simulink model "Computer"  (R2023a)
settings: Solver=VariableStepDiscrete  StartTime=0.0  StopTime=inf  RelTol=1e-3  EnableMultiTasking=on
values from neighbouring files (symbols this model uses):
  RomCode = Preprocessor(RomCode, c)    [ROM.m]
undefined symbols (not defined in the file or in its folder): c, in, RomCodeBreakpoints, RomData, RomDataBreakpoints, UartDataRx, UartDataRx_Active
libraries: Miscellaneous x281, simulink_extras x66, Memory_Blocks_Lib x46, simulink x42, Word_Multiplexers_Lib x31, Decoders_Lib x30, Encoders_Lib x10, Counters_Lib x9, Bit_Multiplexers_Lib x8, Arithmetic_Operations_Lib x5, Bit_Demultiplexers_Lib x4, Garbage x1
(part 5 of 6)

== system Computer/Register Debug ==
  In8 : Inport
  In7 : Inport  Port=2
  In6 : Inport  Port=3
  In5 : Inport  Port=4
  In4 : Inport  Port=5
  In3 : Inport  Port=6
  In2 : Inport  Port=7
  In1 : Inport  Port=8
  Bit to Integer Converter{1..8} (8 alike) : simulink/Logic and Bit Operations/Bit to Integer Converter  nbits=16  bitOrder=MSB first  signedOutputValues=Unsigned  outDtype=uint16  outDtypeSigned=Inherit via internal rule
      settings: LibrarySourceBlock=|
      | commutil2/Bit to Integer
      | Converter
  To Workspace : ToWorkspace  VariableName=gp_reg_00  SampleTime=-1
      settings: MaxDataPoints=1  Save2DSignal=2-D array (concatenate along first dimension)
  To Workspace1 : ToWorkspace  VariableName=gp_reg_01  SampleTime=-1
      settings: MaxDataPoints=1  Save2DSignal=2-D array (concatenate along first dimension)
  To Workspace2 : ToWorkspace  VariableName=gp_reg_02  SampleTime=-1
      settings: MaxDataPoints=1  Save2DSignal=2-D array (concatenate along first dimension)
  To Workspace3 : ToWorkspace  VariableName=gp_reg_03  SampleTime=-1
      settings: MaxDataPoints=1  Save2DSignal=2-D array (concatenate along first dimension)
  To Workspace4 : ToWorkspace  VariableName=gp_reg_04  SampleTime=-1
      settings: MaxDataPoints=1  Save2DSignal=2-D array (concatenate along first dimension)
  To Workspace5 : ToWorkspace  VariableName=gp_reg_05  SampleTime=-1
      settings: MaxDataPoints=1  Save2DSignal=2-D array (concatenate along first dimension)
  To Workspace6 : ToWorkspace  VariableName=gp_reg_06  SampleTime=-1
      settings: MaxDataPoints=1  Save2DSignal=2-D array (concatenate along first dimension)
  To Workspace7 : ToWorkspace  VariableName=gp_reg_07  SampleTime=-1
      settings: MaxDataPoints=1  Save2DSignal=2-D array (concatenate along first dimension)
  wires:
  Bit to Integer Converter1/1 -> To Workspace1/1
  Bit to Integer Converter3/1 -> To Workspace3/1
  Bit to Integer Converter7/1 -> To Workspace7/1
  In8/1 -> Bit to Integer Converter8/1
  Bit to Integer Converter4/1 -> To Workspace4/1
  Bit to Integer Converter5/1 -> To Workspace5/1
  Bit to Integer Converter2/1 -> To Workspace2/1
  Bit to Integer Converter8/1 -> To Workspace/1
  Bit to Integer Converter6/1 -> To Workspace6/1
  In6/1 -> Bit to Integer Converter2/1
  In2/1 -> Bit to Integer Converter6/1
  In5/1 -> Bit to Integer Converter3/1
  In4/1 -> Bit to Integer Converter4/1
  In7/1 -> Bit to Integer Converter1/1
  In1/1 -> Bit to Integer Converter7/1
  In3/1 -> Bit to Integer Converter5/1

== system Computer/Screen_40x25 ==
  Data(1000B) : Inport
  Byte_2 : Constant  Value=c.char_7x7(:, :, 1:256)  OutDataTypeStr=uint8
  MATLAB Function : MATLAB Function  TreatAsAtomicUnit=on
  Matrix Viewer1 : dspobslib/Matrix Viewer  ImageParams=off  CMapStr=[0 0.3 0; 0 1 0]  AxisColorbar=on  AxisParams=off  AxisOrigin=Upper left corner  AxisTickMode=Auto  XTickRange=[0 1]  YTickRange=[0 1]  XLabel=X-axis  YLabel=Y-axis  ZLabel=Z-axis  FigPos=[1280 555 320*2 246*2]  AxisZoom=on
      settings: YMin=0  YMax=1
  wires:
  MATLAB Function/1(Framebuffer) -> Matrix Viewer1/1
  Data(1000B)/1 -> MATLAB Function/2(VideoMemory)
  Byte_2/1 -> MATLAB Function/1(CharTable)

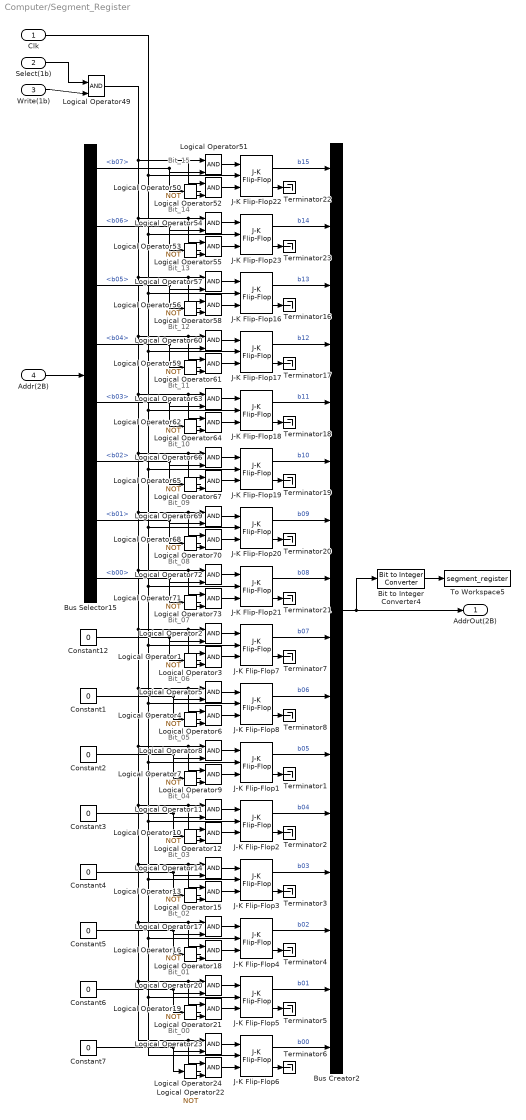
== system Computer/Segment_Register ==
  note: Bit_00
  note: Bit_01
  note: Bit_02
  note: Bit_03
  note: Bit_04
  note: Bit_05
  note: Bit_06
  note: Bit_07
  note: Bit_08
  note: Bit_09
  note: Bit_10
  note: Bit_11
  note: Bit_12
  note: Bit_13
  note: Bit_14
  note: Bit_15
  Clk : Inport  OutDataTypeStr=double
  Select(1b) : Inport  Port=2
  Write(1b) : Inport  Port=3
  Addr(2B) : Inport  Port=4
  Bit to Integer Converter4 : simulink/Logic and Bit Operations/Bit to Integer Converter  nbits=16  bitOrder=MSB first  signedOutputValues=Unsigned  outDtype=uint16  outDtypeSigned=Inherit via internal rule
      settings: LibrarySourceBlock=|
      | commutil2/Bit to Integer
      | Converter
  Bus Creator2 : BusCreator  Inputs=16
  Bus Selector15 : BusSelector  OutputSignals=b07,b06,b05,b04,b03,b02,b01,b00
  Constant{1..7,12} (8 alike) : Constant  Value=0  OutDataTypeStr=boolean
  J-K Flip-Flop{1..8,16..23} (16 alike) : simulink_extras/Flip Flops/J-K Flip-Flop  initial_condition=0
  Logical Operator{1,4,7,10,13,16,19,22,50,53,56,59,62,65,68,71} (16 alike) : Logic  Operator=NOT  IconShape=distinctive  AllPortsSameDT=off  OutDataTypeStr=boolean
  Logical Operator{2..3,5..6,8..9,11..12,14..15,17..18,20..21,23..24,49,51..52,54..55,57..58,60..61,63..64,66..67,69..70,72..73} (33 alike) : Logic  IconShape=distinctive  AllPortsSameDT=off  OutDataTypeStr=boolean
  Terminator{1..8,16..23} (16 alike) : Terminator
  To Workspace5 : ToWorkspace  VariableName=segment_register  SampleTime=-1
      settings: MaxDataPoints=1  Save2DSignal=2-D array (concatenate along first dimension)
  AddrOut(2B) : Outport
  wires:
  J-K Flip-Flop6/2 -> Terminator6/1
  J-K Flip-Flop6/1 -> Bus Creator2/16  "b00"
  Logical Operator22/1 -> Logical Operator24/2
  Logical Operator23/1 -> J-K Flip-Flop6/1
  Logical Operator24/1 -> J-K Flip-Flop6/3
  J-K Flip-Flop5/2 -> Terminator5/1
  J-K Flip-Flop5/1 -> Bus Creator2/15  "b01"
  Logical Operator49/1 -> Logical Operator52/1, Logical Operator51/1, Logical Operator72/1, Logical Operator73/1, Logical Operator20/1, Logical Operator21/1, Logical Operator23/1, Logical Operator24/1, Logical Operator17/1, Logical Operator18/1, Logical Operator14/1, Logical Operator15/1, Logical Operator11/1, Logical Operator12/1, Logical Operator8/1, Logical Operator9/1, Logical Operator5/1, Logical Operator6/1, Logical Operator3/1, Logical Operator2/1, Logical Operator69/1, Logical Operator70/1, Logical Operator66/1, Logical Operator67/1, Logical Operator63/1, Logical Operator64/1, Logical Operator60/1, Logical Operator61/1, Logical Operator57/1, Logical Operator58/1, Logical Operator54/1, Logical Operator55/1
  Logical Operator19/1 -> Logical Operator21/2
  Logical Operator20/1 -> J-K Flip-Flop5/1
  Logical Operator21/1 -> J-K Flip-Flop5/3
  J-K Flip-Flop4/2 -> Terminator4/1
  J-K Flip-Flop4/1 -> Bus Creator2/14  "b02"
  Logical Operator16/1 -> Logical Operator18/2
  Logical Operator17/1 -> J-K Flip-Flop4/1
  Logical Operator18/1 -> J-K Flip-Flop4/3
  J-K Flip-Flop3/2 -> Terminator3/1
  J-K Flip-Flop3/1 -> Bus Creator2/13  "b03"
  Logical Operator13/1 -> Logical Operator15/2
  Logical Operator14/1 -> J-K Flip-Flop3/1
  Logical Operator15/1 -> J-K Flip-Flop3/3
  J-K Flip-Flop2/2 -> Terminator2/1
  J-K Flip-Flop2/1 -> Bus Creator2/12  "b04"
  Logical Operator10/1 -> Logical Operator12/2
  Logical Operator11/1 -> J-K Flip-Flop2/1
  Logical Operator12/1 -> J-K Flip-Flop2/3
  J-K Flip-Flop1/2 -> Terminator1/1
  J-K Flip-Flop1/1 -> Bus Creator2/11  "b05"
  Clk/1 -> J-K Flip-Flop22/2, J-K Flip-Flop23/2, J-K Flip-Flop16/2, J-K Flip-Flop17/2, J-K Flip-Flop18/2, J-K Flip-Flop19/2, J-K Flip-Flop20/2, J-K Flip-Flop21/2, J-K Flip-Flop7/2, J-K Flip-Flop8/2, J-K Flip-Flop2/2, J-K Flip-Flop3/2, J-K Flip-Flop4/2, J-K Flip-Flop5/2, J-K Flip-Flop6/2, J-K Flip-Flop1/2
  Logical Operator7/1 -> Logical Operator9/2
  Logical Operator8/1 -> J-K Flip-Flop1/1
  Logical Operator9/1 -> J-K Flip-Flop1/3
  J-K Flip-Flop8/2 -> Terminator8/1
  J-K Flip-Flop8/1 -> Bus Creator2/10  "b06"
  Logical Operator4/1 -> Logical Operator6/2
  Logical Operator5/1 -> J-K Flip-Flop8/1
  Logical Operator6/1 -> J-K Flip-Flop8/3
  J-K Flip-Flop7/2 -> Terminator7/1
  J-K Flip-Flop7/1 -> Bus Creator2/9  "b07"
  Logical Operator1/1 -> Logical Operator3/2
  Logical Operator2/1 -> J-K Flip-Flop7/1
  Logical Operator3/1 -> J-K Flip-Flop7/3
  Bus Selector15/1 -> Logical Operator50/1, Logical Operator51/2  "<b07>"
  Bus Selector15/8 -> Logical Operator72/2, Logical Operator71/1  "<b00>"
  J-K Flip-Flop21/2 -> Terminator21/1
  J-K Flip-Flop21/1 -> Bus Creator2/8  "b08"
  Logical Operator71/1 -> Logical Operator73/2
  Logical Operator72/1 -> J-K Flip-Flop21/1
  Logical Operator73/1 -> J-K Flip-Flop21/3
  Bus Selector15/7 -> Logical Operator69/2, Logical Operator68/1  "<b01>"
  J-K Flip-Flop20/2 -> Terminator20/1
  J-K Flip-Flop20/1 -> Bus Creator2/7  "b09"
  Logical Operator68/1 -> Logical Operator70/2
  Logical Operator69/1 -> J-K Flip-Flop20/1
  Logical Operator70/1 -> J-K Flip-Flop20/3
  Bus Selector15/6 -> Logical Operator66/2, Logical Operator65/1  "<b02>"
  J-K Flip-Flop19/2 -> Terminator19/1
  J-K Flip-Flop19/1 -> Bus Creator2/6  "b10"
  Logical Operator65/1 -> Logical Operator67/2
  Logical Operator66/1 -> J-K Flip-Flop19/1
  Logical Operator67/1 -> J-K Flip-Flop19/3
  Bus Selector15/5 -> Logical Operator63/2, Logical Operator62/1  "<b03>"
  J-K Flip-Flop18/2 -> Terminator18/1
  J-K Flip-Flop18/1 -> Bus Creator2/5  "b11"
  Logical Operator62/1 -> Logical Operator64/2
  Logical Operator63/1 -> J-K Flip-Flop18/1
  Logical Operator64/1 -> J-K Flip-Flop18/3
  Bus Selector15/4 -> Logical Operator60/2, Logical Operator59/1  "<b04>"
  J-K Flip-Flop17/2 -> Terminator17/1
  J-K Flip-Flop17/1 -> Bus Creator2/4  "b12"
  Logical Operator59/1 -> Logical Operator61/2
  Logical Operator60/1 -> J-K Flip-Flop17/1
  Logical Operator61/1 -> J-K Flip-Flop17/3
  Bus Selector15/3 -> Logical Operator57/2, Logical Operator56/1  "<b05>"
  J-K Flip-Flop16/2 -> Terminator16/1
  J-K Flip-Flop16/1 -> Bus Creator2/3  "b13"
  Logical Operator56/1 -> Logical Operator58/2
  Logical Operator57/1 -> J-K Flip-Flop16/1
  Logical Operator58/1 -> J-K Flip-Flop16/3
  Bus Selector15/2 -> Logical Operator53/1, Logical Operator54/2  "<b06>"
  J-K Flip-Flop23/2 -> Terminator23/1
  J-K Flip-Flop23/1 -> Bus Creator2/2  "b14"
  Logical Operator53/1 -> Logical Operator55/2
  Logical Operator54/1 -> J-K Flip-Flop23/1
  Logical Operator55/1 -> J-K Flip-Flop23/3
  J-K Flip-Flop22/2 -> Terminator22/1
  J-K Flip-Flop22/1 -> Bus Creator2/1  "b15"
  Logical Operator50/1 -> Logical Operator52/2
  Logical Operator51/1 -> J-K Flip-Flop22/1
  Logical Operator52/1 -> J-K Flip-Flop22/3
  Addr(2B)/1 -> Bus Selector15/1
  Select(1b)/1 -> Logical Operator49/1
  Write(1b)/1 -> Logical Operator49/2
  Bus Creator2/1 -> Bit to Integer Converter4/1, AddrOut(2B)/1
  Bit to Integer Converter4/1 -> To Workspace5/1
  Constant12/1 -> Logical Operator1/1, Logical Operator2/2
  Constant1/1 -> Logical Operator4/1, Logical Operator5/2
  Constant2/1 -> Logical Operator8/2, Logical Operator7/1
  Constant3/1 -> Logical Operator10/1, Logical Operator11/2
  Constant4/1 -> Logical Operator13/1, Logical Operator14/2
  Constant5/1 -> Logical Operator17/2, Logical Operator16/1
  Constant6/1 -> Logical Operator20/2, Logical Operator19/1
  Constant7/1 -> Logical Operator22/1, Logical Operator23/2

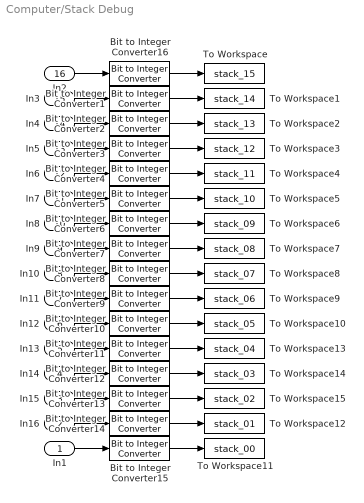
== system Computer/Stack Debug ==
  In1 : Inport
  In16 : Inport  Port=2
  In15 : Inport  Port=3
  In14 : Inport  Port=4
  In13 : Inport  Port=5
  In12 : Inport  Port=6
  In11 : Inport  Port=7
  In10 : Inport  Port=8
  In9 : Inport  Port=9
  In8 : Inport  Port=10
  In7 : Inport  Port=11
  In6 : Inport  Port=12
  In5 : Inport  Port=13
  In4 : Inport  Port=14
  In3 : Inport  Port=15
  In2 : Inport  Port=16
  Bit to Integer Converter{1..16} (16 alike) : simulink/Logic and Bit Operations/Bit to Integer Converter  nbits=16  bitOrder=MSB first  signedOutputValues=Unsigned  outDtype=uint16  outDtypeSigned=Inherit via internal rule
      settings: LibrarySourceBlock=|
      | commutil2/Bit to Integer
      | Converter
  To Workspace : ToWorkspace  VariableName=stack_15  SampleTime=-1
      settings: MaxDataPoints=1  Save2DSignal=2-D array (concatenate along first dimension)
  To Workspace1 : ToWorkspace  VariableName=stack_14  SampleTime=-1
      settings: MaxDataPoints=1  Save2DSignal=2-D array (concatenate along first dimension)
  To Workspace10 : ToWorkspace  VariableName=stack_05  SampleTime=-1
      settings: MaxDataPoints=1  Save2DSignal=2-D array (concatenate along first dimension)
  To Workspace11 : ToWorkspace  VariableName=stack_00  SampleTime=-1
      settings: MaxDataPoints=1  Save2DSignal=2-D array (concatenate along first dimension)
  To Workspace12 : ToWorkspace  VariableName=stack_01  SampleTime=-1
      settings: MaxDataPoints=1  Save2DSignal=2-D array (concatenate along first dimension)
  To Workspace13 : ToWorkspace  VariableName=stack_04  SampleTime=-1
      settings: MaxDataPoints=1  Save2DSignal=2-D array (concatenate along first dimension)
  To Workspace14 : ToWorkspace  VariableName=stack_03  SampleTime=-1
      settings: MaxDataPoints=1  Save2DSignal=2-D array (concatenate along first dimension)
  To Workspace15 : ToWorkspace  VariableName=stack_02  SampleTime=-1
      settings: MaxDataPoints=1  Save2DSignal=2-D array (concatenate along first dimension)
  To Workspace2 : ToWorkspace  VariableName=stack_13  SampleTime=-1
      settings: MaxDataPoints=1  Save2DSignal=2-D array (concatenate along first dimension)
  To Workspace3 : ToWorkspace  VariableName=stack_12  SampleTime=-1
      settings: MaxDataPoints=1  Save2DSignal=2-D array (concatenate along first dimension)
  To Workspace4 : ToWorkspace  VariableName=stack_11  SampleTime=-1
      settings: MaxDataPoints=1  Save2DSignal=2-D array (concatenate along first dimension)
  To Workspace5 : ToWorkspace  VariableName=stack_10  SampleTime=-1
      settings: MaxDataPoints=1  Save2DSignal=2-D array (concatenate along first dimension)
  To Workspace6 : ToWorkspace  VariableName=stack_09  SampleTime=-1
      settings: MaxDataPoints=1  Save2DSignal=2-D array (concatenate along first dimension)
  To Workspace7 : ToWorkspace  VariableName=stack_08  SampleTime=-1
      settings: MaxDataPoints=1  Save2DSignal=2-D array (concatenate along first dimension)
  To Workspace8 : ToWorkspace  VariableName=stack_07  SampleTime=-1
      settings: MaxDataPoints=1  Save2DSignal=2-D array (concatenate along first dimension)
  To Workspace9 : ToWorkspace  VariableName=stack_06  SampleTime=-1
      settings: MaxDataPoints=1  Save2DSignal=2-D array (concatenate along first dimension)
  wires:
  Bit to Integer Converter8/1 -> To Workspace8/1
  Bit to Integer Converter2/1 -> To Workspace2/1
  Bit to Integer Converter13/1 -> To Workspace15/1
  In5/1 -> Bit to Integer Converter3/1
  Bit to Integer Converter3/1 -> To Workspace3/1
  Bit to Integer Converter6/1 -> To Workspace6/1
  In3/1 -> Bit to Integer Converter1/1
  Bit to Integer Converter12/1 -> To Workspace14/1
  Bit to Integer Converter5/1 -> To Workspace5/1
  Bit to Integer Converter15/1 -> To Workspace11/1
  Bit to Integer Converter11/1 -> To Workspace13/1
  In16/1 -> Bit to Integer Converter14/1
  Bit to Integer Converter10/1 -> To Workspace10/1
  Bit to Integer Converter7/1 -> To Workspace7/1
  Bit to Integer Converter14/1 -> To Workspace12/1
  In10/1 -> Bit to Integer Converter8/1
  Bit to Integer Converter9/1 -> To Workspace9/1
  Bit to Integer Converter4/1 -> To Workspace4/1
  Bit to Integer Converter16/1 -> To Workspace/1
  Bit to Integer Converter1/1 -> To Workspace1/1
  In9/1 -> Bit to Integer Converter7/1
  In11/1 -> Bit to Integer Converter9/1
  In12/1 -> Bit to Integer Converter10/1
  In13/1 -> Bit to Integer Converter11/1
  In14/1 -> Bit to Integer Converter12/1
  In1/1 -> Bit to Integer Converter15/1
  In8/1 -> Bit to Integer Converter6/1
  In7/1 -> Bit to Integer Converter5/1
  In6/1 -> Bit to Integer Converter4/1
  In15/1 -> Bit to Integer Converter13/1
  In2/1 -> Bit to Integer Converter16/1
  In4/1 -> Bit to Integer Converter2/1

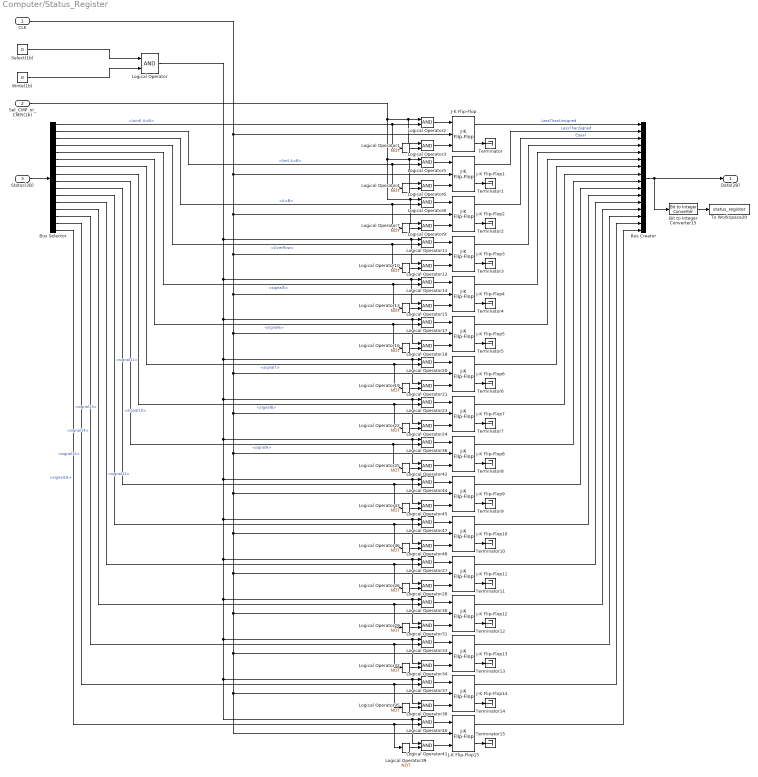
== system Computer/Status_Register ==
  CLK : Inport  OutDataTypeStr=double
  Sel_CMP_or_CMPI(1b) : Inport  Port=2
  Status(2B) : Inport  Port=3
  Bit to Integer Converter15 : simulink/Logic and Bit Operations/Bit to Integer Converter  nbits=16  bitOrder=MSB first  signedOutputValues=Unsigned  outDtype=uint16  outDtypeSigned=Inherit via internal rule
      settings: LibrarySourceBlock=|
      | commutil2/Bit to Integer
      | Converter
  Bus Creator : BusCreator  Inputs=16
  Bus Selector : BusSelector  OutputSignals=(uint) A<B,(int) A<B,A=B,Overflow,signal5,signal6,signal7,signal8,signal9,signal10,signal11,signal12,signal13,signal14,signal15,signal16
  J-K Flip-Flop{,1..15} (16 alike) : simulink_extras/Flip Flops/J-K Flip-Flop  initial_condition=0
  Logical Operator{,2..3,5..6,8..9,11..12,14..15,17..18,20..21,23..24,27..28,30..31,33..34,36..38,40..42,44..45,47..48} (33 alike) : Logic  IconShape=distinctive  AllPortsSameDT=off  OutDataTypeStr=boolean
  Logical Operator{1,4,7,10,13,16,19,22,25..26,29,32,35,39,43,46} (16 alike) : Logic  Operator=NOT  IconShape=distinctive  AllPortsSameDT=off  OutDataTypeStr=boolean
  Select(1b) : Constant  Value=0  OutDataTypeStr=boolean
  Terminator{,1..15} (16 alike) : Terminator
  To Workspace20 : ToWorkspace  VariableName=status_register  SampleTime=-1
      settings: MaxDataPoints=1  Save2DSignal=2-D array (concatenate along first dimension)
  Write(1b) : Constant  Value=0  OutDataTypeStr=boolean
  Data(2B) : Outport
  wires:
  Logical Operator41/1 -> J-K Flip-Flop15/3
  Logical Operator40/1 -> J-K Flip-Flop15/1
  Logical Operator39/1 -> Logical Operator41/2
  Logical Operator/1 -> Logical Operator11/1, Logical Operator12/1, Logical Operator14/1, Logical Operator15/1, Logical Operator18/1, Logical Operator17/1, Logical Operator20/1, Logical Operator21/1, Logical Operator23/1, Logical Operator24/1, Logical Operator36/1, Logical Operator42/1, Logical Operator44/1, Logical Operator45/1, Logical Operator47/1, Logical Operator48/1, Logical Operator27/1, Logical Operator28/1, Logical Operator30/1, Logical Operator31/1, Logical Operator34/1, Logical Operator33/1, Logical Operator37/1, Logical Operator38/1, Logical Operator40/1, Logical Operator41/1
  CLK/1 -> J-K Flip-Flop/2, J-K Flip-Flop1/2, J-K Flip-Flop2/2, J-K Flip-Flop3/2, J-K Flip-Flop4/2, J-K Flip-Flop5/2, J-K Flip-Flop7/2, J-K Flip-Flop8/2, J-K Flip-Flop9/2, J-K Flip-Flop10/2, J-K Flip-Flop11/2, J-K Flip-Flop12/2, J-K Flip-Flop13/2, J-K Flip-Flop15/2, J-K Flip-Flop14/2, J-K Flip-Flop6/2
  J-K Flip-Flop15/2 -> Terminator15/1
  Bus Selector/16 -> Logical Operator40/2, Logical Operator39/1  "<signal16>"
  Logical Operator38/1 -> J-K Flip-Flop14/3
  Logical Operator37/1 -> J-K Flip-Flop14/1
  Logical Operator35/1 -> Logical Operator38/2
  J-K Flip-Flop14/2 -> Terminator14/1
  Bus Selector/15 -> Logical Operator37/2, Logical Operator35/1  "<signal15>"
  Logical Operator34/1 -> J-K Flip-Flop13/3
  Logical Operator33/1 -> J-K Flip-Flop13/1
  Logical Operator32/1 -> Logical Operator34/2
  J-K Flip-Flop13/2 -> Terminator13/1
  Bus Selector/14 -> Logical Operator32/1, Logical Operator33/2  "<signal14>"
  Logical Operator31/1 -> J-K Flip-Flop12/3
  Logical Operator30/1 -> J-K Flip-Flop12/1
  Logical Operator29/1 -> Logical Operator31/2
  J-K Flip-Flop12/2 -> Terminator12/1
  Bus Selector/13 -> Logical Operator30/2, Logical Operator29/1  "<signal13>"
  Logical Operator28/1 -> J-K Flip-Flop11/3
  Logical Operator27/1 -> J-K Flip-Flop11/1
  Logical Operator26/1 -> Logical Operator28/2
  J-K Flip-Flop11/2 -> Terminator11/1
  Bus Selector/12 -> Logical Operator26/1, Logical Operator27/2  "<signal12>"
  Logical Operator48/1 -> J-K Flip-Flop10/3
  Logical Operator47/1 -> J-K Flip-Flop10/1
  Logical Operator46/1 -> Logical Operator48/2
  J-K Flip-Flop10/2 -> Terminator10/1
  Bus Selector/11 -> Logical Operator47/2, Logical Operator46/1  "<signal11>"
  Logical Operator45/1 -> J-K Flip-Flop9/3
  Logical Operator44/1 -> J-K Flip-Flop9/1
  Logical Operator43/1 -> Logical Operator45/2
  J-K Flip-Flop9/2 -> Terminator9/1
  Bus Selector/10 -> Logical Operator44/2, Logical Operator43/1  "<signal10>"
  Logical Operator42/1 -> J-K Flip-Flop8/3
  Logical Operator36/1 -> J-K Flip-Flop8/1
  Logical Operator25/1 -> Logical Operator42/2
  J-K Flip-Flop8/2 -> Terminator8/1
  Bus Selector/9 -> Logical Operator36/2, Logical Operator25/1  "<signal9>"
  J-K Flip-Flop8/1 -> Bus Creator/9
  J-K Flip-Flop9/1 -> Bus Creator/10
  J-K Flip-Flop10/1 -> Bus Creator/11
  J-K Flip-Flop11/1 -> Bus Creator/12
  J-K Flip-Flop12/1 -> Bus Creator/13
  J-K Flip-Flop13/1 -> Bus Creator/14
  J-K Flip-Flop14/1 -> Bus Creator/15
  J-K Flip-Flop15/1 -> Bus Creator/16
  Logical Operator24/1 -> J-K Flip-Flop7/3
  Logical Operator23/1 -> J-K Flip-Flop7/1
  Logical Operator22/1 -> Logical Operator24/2
  J-K Flip-Flop7/2 -> Terminator7/1
  Bus Selector/8 -> Logical Operator23/2, Logical Operator22/1  "<signal8>"
  Logical Operator21/1 -> J-K Flip-Flop6/3
  Logical Operator20/1 -> J-K Flip-Flop6/1
  Logical Operator19/1 -> Logical Operator21/2
  J-K Flip-Flop6/2 -> Terminator6/1
  Bus Selector/7 -> Logical Operator20/2, Logical Operator19/1  "<signal7>"
  Logical Operator18/1 -> J-K Flip-Flop5/3
  Logical Operator17/1 -> J-K Flip-Flop5/1
  Logical Operator16/1 -> Logical Operator18/2
  J-K Flip-Flop5/2 -> Terminator5/1
  Bus Selector/6 -> Logical Operator16/1, Logical Operator17/2  "<signal6>"
  Logical Operator15/1 -> J-K Flip-Flop4/3
  Logical Operator14/1 -> J-K Flip-Flop4/1
  Logical Operator13/1 -> Logical Operator15/2
  J-K Flip-Flop4/2 -> Terminator4/1
  Bus Selector/5 -> Logical Operator13/1, Logical Operator14/2  "<signal5>"
  Logical Operator12/1 -> J-K Flip-Flop3/3
  Logical Operator11/1 -> J-K Flip-Flop3/1
  Logical Operator10/1 -> Logical Operator12/2
  J-K Flip-Flop3/2 -> Terminator3/1
  Bus Selector/4 -> Logical Operator10/1, Logical Operator11/2  "<Overflow>"
  Logical Operator9/1 -> J-K Flip-Flop2/3
  Logical Operator8/1 -> J-K Flip-Flop2/1
  Logical Operator7/1 -> Logical Operator9/2
  J-K Flip-Flop2/2 -> Terminator2/1
  Bus Selector/3 -> Logical Operator7/1, Logical Operator8/2  "<A=B>"
  Logical Operator6/1 -> J-K Flip-Flop1/3
  Logical Operator5/1 -> J-K Flip-Flop1/1
  Logical Operator4/1 -> Logical Operator6/2
  J-K Flip-Flop1/2 -> Terminator1/1
  Bus Selector/2 -> Logical Operator5/2, Logical Operator4/1  "<(int) A<B>"
  Logical Operator3/1 -> J-K Flip-Flop/3
  Logical Operator2/1 -> J-K Flip-Flop/1
  Logical Operator1/1 -> Logical Operator3/2
  J-K Flip-Flop/2 -> Terminator/1
  Bus Selector/1 -> Logical Operator2/2, Logical Operator1/1  "<(uint) A<B>"
  Bus Creator/1 -> Bit to Integer Converter15/1, Data(2B)/1
  J-K Flip-Flop/1 -> Bus Creator/1  "LessThanUnsigned"
  J-K Flip-Flop1/1 -> Bus Creator/2  "LessThanSigned"
  J-K Flip-Flop2/1 -> Bus Creator/3  "Equal"
  J-K Flip-Flop3/1 -> Bus Creator/4
  J-K Flip-Flop4/1 -> Bus Creator/5
  J-K Flip-Flop5/1 -> Bus Creator/6
  J-K Flip-Flop6/1 -> Bus Creator/7
  J-K Flip-Flop7/1 -> Bus Creator/8
  Select(1b)/1 -> Logical Operator/1
  Write(1b)/1 -> Logical Operator/2
  Sel_CMP_or_CMPI(1b)/1 -> Logical Operator8/1, Logical Operator9/1, Logical Operator5/1, Logical Operator6/1, Logical Operator2/1, Logical Operator3/1
  Status(2B)/1 -> Bus Selector/1
  Bit to Integer Converter15/1 -> To Workspace20/1

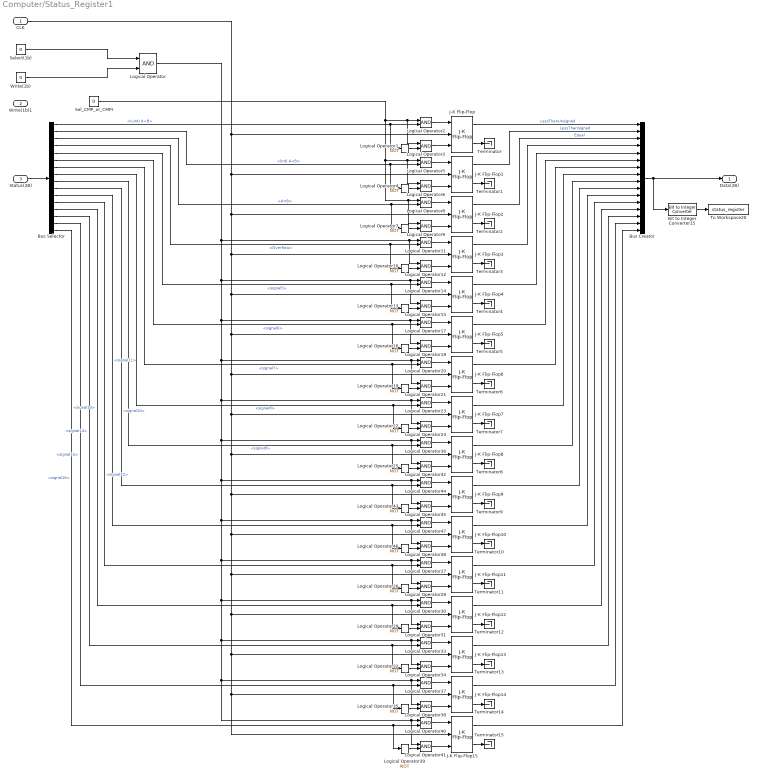
== system Computer/Status_Register1 ==
  CLK : Inport  OutDataTypeStr=double
  Write(1b)1 : Inport  Port=2
  Status(2B) : Inport  Port=3
  Bit to Integer Converter15 : simulink/Logic and Bit Operations/Bit to Integer Converter  nbits=16  bitOrder=MSB first  signedOutputValues=Unsigned  outDtype=uint16  outDtypeSigned=Inherit via internal rule
      settings: LibrarySourceBlock=|
      | commutil2/Bit to Integer
      | Converter
  Bus Creator : BusCreator  Inputs=16
  Bus Selector : BusSelector  OutputSignals=(uint) A<B,(int) A<B,A=B,Overflow,signal5,signal6,signal7,signal8,signal9,signal10,signal11,signal12,signal13,signal14,signal15,signal16
  J-K Flip-Flop{,1..15} (16 alike) : simulink_extras/Flip Flops/J-K Flip-Flop  initial_condition=0
  Logical Operator{,2..3,5..6,8..9,11..12,14..15,17..18,20..21,23..24,27..28,30..31,33..34,36..38,40..42,44..45,47..48} (33 alike) : Logic  IconShape=distinctive  AllPortsSameDT=off  OutDataTypeStr=boolean
  Logical Operator{1,4,7,10,13,16,19,22,25..26,29,32,35,39,43,46} (16 alike) : Logic  Operator=NOT  IconShape=distinctive  AllPortsSameDT=off  OutDataTypeStr=boolean
  Sel_CMP_or_CMPI : Constant  Value=0  OutDataTypeStr=boolean
  Select(1b) : Constant  Value=0  OutDataTypeStr=boolean
  Terminator{,1..15} (16 alike) : Terminator
  To Workspace20 : ToWorkspace  VariableName=status_register  SampleTime=-1
      settings: MaxDataPoints=1  Save2DSignal=2-D array (concatenate along first dimension)
  Write(1b) : Constant  Value=0  OutDataTypeStr=boolean
  Data(2B) : Outport
  wires:
  Logical Operator41/1 -> J-K Flip-Flop15/3
  Logical Operator40/1 -> J-K Flip-Flop15/1
  Logical Operator39/1 -> Logical Operator41/2
  Logical Operator/1 -> Logical Operator11/1, Logical Operator12/1, Logical Operator14/1, Logical Operator15/1, Logical Operator18/1, Logical Operator17/1, Logical Operator20/1, Logical Operator21/1, Logical Operator23/1, Logical Operator24/1, Logical Operator36/1, Logical Operator42/1, Logical Operator44/1, Logical Operator45/1, Logical Operator47/1, Logical Operator48/1, Logical Operator27/1, Logical Operator28/1, Logical Operator30/1, Logical Operator31/1, Logical Operator34/1, Logical Operator33/1, Logical Operator37/1, Logical Operator38/1, Logical Operator40/1, Logical Operator41/1
  CLK/1 -> J-K Flip-Flop/2, J-K Flip-Flop1/2, J-K Flip-Flop2/2, J-K Flip-Flop3/2, J-K Flip-Flop4/2, J-K Flip-Flop5/2, J-K Flip-Flop7/2, J-K Flip-Flop8/2, J-K Flip-Flop9/2, J-K Flip-Flop10/2, J-K Flip-Flop11/2, J-K Flip-Flop12/2, J-K Flip-Flop13/2, J-K Flip-Flop15/2, J-K Flip-Flop14/2, J-K Flip-Flop6/2
  J-K Flip-Flop15/2 -> Terminator15/1
  Bus Selector/16 -> Logical Operator40/2, Logical Operator39/1  "<signal16>"
  Logical Operator38/1 -> J-K Flip-Flop14/3
  Logical Operator37/1 -> J-K Flip-Flop14/1
  Logical Operator35/1 -> Logical Operator38/2
  J-K Flip-Flop14/2 -> Terminator14/1
  Bus Selector/15 -> Logical Operator37/2, Logical Operator35/1  "<signal15>"
  Logical Operator34/1 -> J-K Flip-Flop13/3
  Logical Operator33/1 -> J-K Flip-Flop13/1
  Logical Operator32/1 -> Logical Operator34/2
  J-K Flip-Flop13/2 -> Terminator13/1
  Bus Selector/14 -> Logical Operator32/1, Logical Operator33/2  "<signal14>"
  Logical Operator31/1 -> J-K Flip-Flop12/3
  Logical Operator30/1 -> J-K Flip-Flop12/1
  Logical Operator29/1 -> Logical Operator31/2
  J-K Flip-Flop12/2 -> Terminator12/1
  Bus Selector/13 -> Logical Operator30/2, Logical Operator29/1  "<signal13>"
  Logical Operator28/1 -> J-K Flip-Flop11/3
  Logical Operator27/1 -> J-K Flip-Flop11/1
  Logical Operator26/1 -> Logical Operator28/2
  J-K Flip-Flop11/2 -> Terminator11/1
  Bus Selector/12 -> Logical Operator26/1, Logical Operator27/2  "<signal12>"
  Logical Operator48/1 -> J-K Flip-Flop10/3
  Logical Operator47/1 -> J-K Flip-Flop10/1
  Logical Operator46/1 -> Logical Operator48/2
  J-K Flip-Flop10/2 -> Terminator10/1
  Bus Selector/11 -> Logical Operator47/2, Logical Operator46/1  "<signal11>"
  Logical Operator45/1 -> J-K Flip-Flop9/3
  Logical Operator44/1 -> J-K Flip-Flop9/1
  Logical Operator43/1 -> Logical Operator45/2
  J-K Flip-Flop9/2 -> Terminator9/1
  Bus Selector/10 -> Logical Operator44/2, Logical Operator43/1  "<signal10>"
  Logical Operator42/1 -> J-K Flip-Flop8/3
  Logical Operator36/1 -> J-K Flip-Flop8/1
  Logical Operator25/1 -> Logical Operator42/2
  J-K Flip-Flop8/2 -> Terminator8/1
  Bus Selector/9 -> Logical Operator36/2, Logical Operator25/1  "<signal9>"
  J-K Flip-Flop8/1 -> Bus Creator/9
  J-K Flip-Flop9/1 -> Bus Creator/10
  J-K Flip-Flop10/1 -> Bus Creator/11
  J-K Flip-Flop11/1 -> Bus Creator/12
  J-K Flip-Flop12/1 -> Bus Creator/13
  J-K Flip-Flop13/1 -> Bus Creator/14
  J-K Flip-Flop14/1 -> Bus Creator/15
  J-K Flip-Flop15/1 -> Bus Creator/16
  Logical Operator24/1 -> J-K Flip-Flop7/3
  Logical Operator23/1 -> J-K Flip-Flop7/1
  Logical Operator22/1 -> Logical Operator24/2
  J-K Flip-Flop7/2 -> Terminator7/1
  Bus Selector/8 -> Logical Operator23/2, Logical Operator22/1  "<signal8>"
  Logical Operator21/1 -> J-K Flip-Flop6/3
  Logical Operator20/1 -> J-K Flip-Flop6/1
  Logical Operator19/1 -> Logical Operator21/2
  J-K Flip-Flop6/2 -> Terminator6/1
  Bus Selector/7 -> Logical Operator20/2, Logical Operator19/1  "<signal7>"
  Logical Operator18/1 -> J-K Flip-Flop5/3
  Logical Operator17/1 -> J-K Flip-Flop5/1
  Logical Operator16/1 -> Logical Operator18/2
  J-K Flip-Flop5/2 -> Terminator5/1
  Bus Selector/6 -> Logical Operator16/1, Logical Operator17/2  "<signal6>"
  Logical Operator15/1 -> J-K Flip-Flop4/3
  Logical Operator14/1 -> J-K Flip-Flop4/1
  Logical Operator13/1 -> Logical Operator15/2
  J-K Flip-Flop4/2 -> Terminator4/1
  Bus Selector/5 -> Logical Operator13/1, Logical Operator14/2  "<signal5>"
  Logical Operator12/1 -> J-K Flip-Flop3/3
  Logical Operator11/1 -> J-K Flip-Flop3/1
  Logical Operator10/1 -> Logical Operator12/2
  J-K Flip-Flop3/2 -> Terminator3/1
  Bus Selector/4 -> Logical Operator10/1, Logical Operator11/2  "<Overflow>"
  Logical Operator9/1 -> J-K Flip-Flop2/3
  Logical Operator8/1 -> J-K Flip-Flop2/1
  Logical Operator7/1 -> Logical Operator9/2
  J-K Flip-Flop2/2 -> Terminator2/1
  Bus Selector/3 -> Logical Operator7/1, Logical Operator8/2  "<A=B>"
  Logical Operator6/1 -> J-K Flip-Flop1/3
  Logical Operator5/1 -> J-K Flip-Flop1/1
  Logical Operator4/1 -> Logical Operator6/2
  J-K Flip-Flop1/2 -> Terminator1/1
  Bus Selector/2 -> Logical Operator5/2, Logical Operator4/1  "<(int) A<B>"
  Logical Operator3/1 -> J-K Flip-Flop/3
  Logical Operator2/1 -> J-K Flip-Flop/1
  Logical Operator1/1 -> Logical Operator3/2
  J-K Flip-Flop/2 -> Terminator/1
  Bus Selector/1 -> Logical Operator2/2, Logical Operator1/1  "<(uint) A<B>"
  Bus Creator/1 -> Bit to Integer Converter15/1, Data(2B)/1
  J-K Flip-Flop/1 -> Bus Creator/1  "LessThanUnsigned"
  J-K Flip-Flop1/1 -> Bus Creator/2  "LessThanSigned"
  J-K Flip-Flop2/1 -> Bus Creator/3  "Equal"
  J-K Flip-Flop3/1 -> Bus Creator/4
  J-K Flip-Flop4/1 -> Bus Creator/5
  J-K Flip-Flop5/1 -> Bus Creator/6
  J-K Flip-Flop6/1 -> Bus Creator/7
  J-K Flip-Flop7/1 -> Bus Creator/8
  Select(1b)/1 -> Logical Operator/1
  Write(1b)/1 -> Logical Operator/2
  Sel_CMP_or_CMPI/1 -> Logical Operator8/1, Logical Operator9/1, Logical Operator5/1, Logical Operator6/1, Logical Operator2/1, Logical Operator3/1
  Status(2B)/1 -> Bus Selector/1
  Bit to Integer Converter15/1 -> To Workspace20/1

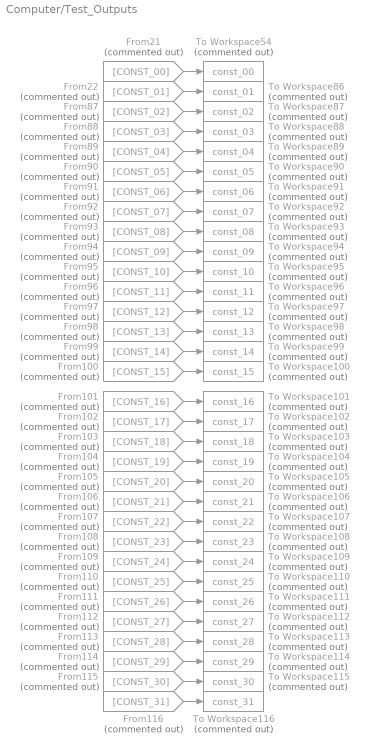
== system Computer/Test_Outputs ==
  From100 : From  Commented=on  GotoTag=CONST_15
  From101 : From  Commented=on  GotoTag=CONST_16
  From102 : From  Commented=on  GotoTag=CONST_17
  From103 : From  Commented=on  GotoTag=CONST_18
  From104 : From  Commented=on  GotoTag=CONST_19
  From105 : From  Commented=on  GotoTag=CONST_20
  From106 : From  Commented=on  GotoTag=CONST_21
  From107 : From  Commented=on  GotoTag=CONST_22
  From108 : From  Commented=on  GotoTag=CONST_23
  From109 : From  Commented=on  GotoTag=CONST_24
  From110 : From  Commented=on  GotoTag=CONST_25
  From111 : From  Commented=on  GotoTag=CONST_26
  From112 : From  Commented=on  GotoTag=CONST_27
  From113 : From  Commented=on  GotoTag=CONST_28
  From114 : From  Commented=on  GotoTag=CONST_29
  From115 : From  Commented=on  GotoTag=CONST_30
  From116 : From  Commented=on  GotoTag=CONST_31
  From21 : From  Commented=on  GotoTag=CONST_00
  From22 : From  Commented=on  GotoTag=CONST_01
  From87 : From  Commented=on  GotoTag=CONST_02
  From88 : From  Commented=on  GotoTag=CONST_03
  From89 : From  Commented=on  GotoTag=CONST_04
  From90 : From  Commented=on  GotoTag=CONST_05
  From91 : From  Commented=on  GotoTag=CONST_06
  From92 : From  Commented=on  GotoTag=CONST_07
  From93 : From  Commented=on  GotoTag=CONST_08
  From94 : From  Commented=on  GotoTag=CONST_09
  From95 : From  Commented=on  GotoTag=CONST_10
  From96 : From  Commented=on  GotoTag=CONST_11
  From97 : From  Commented=on  GotoTag=CONST_12
  From98 : From  Commented=on  GotoTag=CONST_13
  From99 : From  Commented=on  GotoTag=CONST_14
  To Workspace100 : ToWorkspace  Commented=on  VariableName=const_15  SampleTime=-1
      settings: MaxDataPoints=1  Save2DSignal=2-D array (concatenate along first dimension)
  To Workspace101 : ToWorkspace  Commented=on  VariableName=const_16  SampleTime=-1
      settings: MaxDataPoints=1  Save2DSignal=2-D array (concatenate along first dimension)
  To Workspace102 : ToWorkspace  Commented=on  VariableName=const_17  SampleTime=-1
      settings: MaxDataPoints=1  Save2DSignal=2-D array (concatenate along first dimension)
  To Workspace103 : ToWorkspace  Commented=on  VariableName=const_18  SampleTime=-1
      settings: MaxDataPoints=1  Save2DSignal=2-D array (concatenate along first dimension)
  To Workspace104 : ToWorkspace  Commented=on  VariableName=const_19  SampleTime=-1
      settings: MaxDataPoints=1  Save2DSignal=2-D array (concatenate along first dimension)
  To Workspace105 : ToWorkspace  Commented=on  VariableName=const_20  SampleTime=-1
      settings: MaxDataPoints=1  Save2DSignal=2-D array (concatenate along first dimension)
  To Workspace106 : ToWorkspace  Commented=on  VariableName=const_21  SampleTime=-1
      settings: MaxDataPoints=1  Save2DSignal=2-D array (concatenate along first dimension)
  To Workspace107 : ToWorkspace  Commented=on  VariableName=const_22  SampleTime=-1
      settings: MaxDataPoints=1  Save2DSignal=2-D array (concatenate along first dimension)
  To Workspace108 : ToWorkspace  Commented=on  VariableName=const_23  SampleTime=-1
      settings: MaxDataPoints=1  Save2DSignal=2-D array (concatenate along first dimension)
  To Workspace109 : ToWorkspace  Commented=on  VariableName=const_24  SampleTime=-1
      settings: MaxDataPoints=1  Save2DSignal=2-D array (concatenate along first dimension)
  To Workspace110 : ToWorkspace  Commented=on  VariableName=const_25  SampleTime=-1
      settings: MaxDataPoints=1  Save2DSignal=2-D array (concatenate along first dimension)
  To Workspace111 : ToWorkspace  Commented=on  VariableName=const_26  SampleTime=-1
      settings: MaxDataPoints=1  Save2DSignal=2-D array (concatenate along first dimension)
  To Workspace112 : ToWorkspace  Commented=on  VariableName=const_27  SampleTime=-1
      settings: MaxDataPoints=1  Save2DSignal=2-D array (concatenate along first dimension)
  To Workspace113 : ToWorkspace  Commented=on  VariableName=const_28  SampleTime=-1
      settings: MaxDataPoints=1  Save2DSignal=2-D array (concatenate along first dimension)
  To Workspace114 : ToWorkspace  Commented=on  VariableName=const_29  SampleTime=-1
      settings: MaxDataPoints=1  Save2DSignal=2-D array (concatenate along first dimension)
  To Workspace115 : ToWorkspace  Commented=on  VariableName=const_30  SampleTime=-1
      settings: MaxDataPoints=1  Save2DSignal=2-D array (concatenate along first dimension)
  To Workspace116 : ToWorkspace  Commented=on  VariableName=const_31  SampleTime=-1
      settings: MaxDataPoints=1  Save2DSignal=2-D array (concatenate along first dimension)
  To Workspace54 : ToWorkspace  Commented=on  VariableName=const_00  SampleTime=-1
      settings: MaxDataPoints=1  Save2DSignal=2-D array (concatenate along first dimension)
  To Workspace86 : ToWorkspace  Commented=on  VariableName=const_01  SampleTime=-1
      settings: MaxDataPoints=1  Save2DSignal=2-D array (concatenate along first dimension)
  To Workspace87 : ToWorkspace  Commented=on  VariableName=const_02  SampleTime=-1
      settings: MaxDataPoints=1  Save2DSignal=2-D array (concatenate along first dimension)
  To Workspace88 : ToWorkspace  Commented=on  VariableName=const_03  SampleTime=-1
      settings: MaxDataPoints=1  Save2DSignal=2-D array (concatenate along first dimension)
  To Workspace89 : ToWorkspace  Commented=on  VariableName=const_04  SampleTime=-1
      settings: MaxDataPoints=1  Save2DSignal=2-D array (concatenate along first dimension)
  To Workspace90 : ToWorkspace  Commented=on  VariableName=const_05  SampleTime=-1
      settings: MaxDataPoints=1  Save2DSignal=2-D array (concatenate along first dimension)
  To Workspace91 : ToWorkspace  Commented=on  VariableName=const_06  SampleTime=-1
      settings: MaxDataPoints=1  Save2DSignal=2-D array (concatenate along first dimension)
  To Workspace92 : ToWorkspace  Commented=on  VariableName=const_07  SampleTime=-1
      settings: MaxDataPoints=1  Save2DSignal=2-D array (concatenate along first dimension)
  To Workspace93 : ToWorkspace  Commented=on  VariableName=const_08  SampleTime=-1
      settings: MaxDataPoints=1  Save2DSignal=2-D array (concatenate along first dimension)
  To Workspace94 : ToWorkspace  Commented=on  VariableName=const_09  SampleTime=-1
      settings: MaxDataPoints=1  Save2DSignal=2-D array (concatenate along first dimension)
  To Workspace95 : ToWorkspace  Commented=on  VariableName=const_10  SampleTime=-1
      settings: MaxDataPoints=1  Save2DSignal=2-D array (concatenate along first dimension)
  To Workspace96 : ToWorkspace  Commented=on  VariableName=const_11  SampleTime=-1
      settings: MaxDataPoints=1  Save2DSignal=2-D array (concatenate along first dimension)
  To Workspace97 : ToWorkspace  Commented=on  VariableName=const_12  SampleTime=-1
      settings: MaxDataPoints=1  Save2DSignal=2-D array (concatenate along first dimension)
  To Workspace98 : ToWorkspace  Commented=on  VariableName=const_13  SampleTime=-1
      settings: MaxDataPoints=1  Save2DSignal=2-D array (concatenate along first dimension)
  To Workspace99 : ToWorkspace  Commented=on  VariableName=const_14  SampleTime=-1
      settings: MaxDataPoints=1  Save2DSignal=2-D array (concatenate along first dimension)
  wires:
  From21/1 -> To Workspace54/1
  From22/1 -> To Workspace86/1
  From87/1 -> To Workspace87/1
  From88/1 -> To Workspace88/1
  From89/1 -> To Workspace89/1
  From90/1 -> To Workspace90/1
  From91/1 -> To Workspace91/1
  From92/1 -> To Workspace92/1
  From93/1 -> To Workspace93/1
  From94/1 -> To Workspace94/1
  From95/1 -> To Workspace95/1
  From96/1 -> To Workspace96/1
  From97/1 -> To Workspace97/1
  From98/1 -> To Workspace98/1
  From99/1 -> To Workspace99/1
  From100/1 -> To Workspace100/1
  From101/1 -> To Workspace101/1
  From102/1 -> To Workspace102/1
  From103/1 -> To Workspace103/1
  From104/1 -> To Workspace104/1
  From105/1 -> To Workspace105/1
  From106/1 -> To Workspace106/1
  From108/1 -> To Workspace108/1
  From109/1 -> To Workspace109/1
  From110/1 -> To Workspace110/1
  From107/1 -> To Workspace107/1
  From111/1 -> To Workspace111/1
  From112/1 -> To Workspace112/1
  From113/1 -> To Workspace113/1
  From114/1 -> To Workspace114/1
  From115/1 -> To Workspace115/1
  From116/1 -> To Workspace116/1

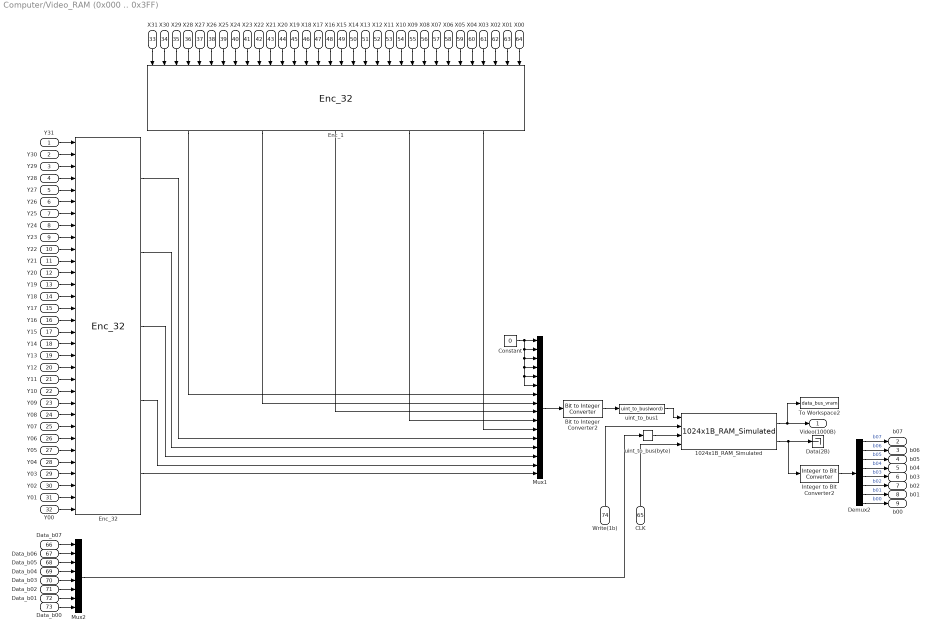
== system Computer/Video_RAM (0x000 .. 0x3FF) ==
  Y31 : Inport
  Y30 : Inport  Port=2
  Y29 : Inport  Port=3
  Y28 : Inport  Port=4
  Y27 : Inport  Port=5
  Y26 : Inport  Port=6
  Y25 : Inport  Port=7
  Y24 : Inport  Port=8
  Y23 : Inport  Port=9
  Y22 : Inport  Port=10
  Y21 : Inport  Port=11
  Y20 : Inport  Port=12
  Y19 : Inport  Port=13
  Y18 : Inport  Port=14
  Y17 : Inport  Port=15
  Y16 : Inport  Port=16
  Y15 : Inport  Port=17
  Y14 : Inport  Port=18
  Y13 : Inport  Port=19
  Y12 : Inport  Port=20
  Y11 : Inport  Port=21
  Y10 : Inport  Port=22
  Y09 : Inport  Port=23
  Y08 : Inport  Port=24
  Y07 : Inport  Port=25
  Y06 : Inport  Port=26
  Y05 : Inport  Port=27
  Y04 : Inport  Port=28
  Y03 : Inport  Port=29
  Y02 : Inport  Port=30
  Y01 : Inport  Port=31
  Y00 : Inport  Port=32
  X31 : Inport  Port=33
  X30 : Inport  Port=34
  X29 : Inport  Port=35
  X28 : Inport  Port=36
  X27 : Inport  Port=37
  X26 : Inport  Port=38
  X25 : Inport  Port=39
  X24 : Inport  Port=40
  X23 : Inport  Port=41
  X22 : Inport  Port=42
  X21 : Inport  Port=43
  X20 : Inport  Port=44
  X19 : Inport  Port=45
  X18 : Inport  Port=46
  X17 : Inport  Port=47
  X16 : Inport  Port=48
  X15 : Inport  Port=49
  X14 : Inport  Port=50
  X13 : Inport  Port=51
  X12 : Inport  Port=52
  X11 : Inport  Port=53
  X10 : Inport  Port=54
  X09 : Inport  Port=55
  X08 : Inport  Port=56
  X07 : Inport  Port=57
  X06 : Inport  Port=58
  X05 : Inport  Port=59
  X04 : Inport  Port=60
  X03 : Inport  Port=61
  X02 : Inport  Port=62
  X01 : Inport  Port=63
  X00 : Inport  Port=64
  CLK : Inport  Port=65
  Data_b07 : Inport  Port=66
  Data_b06 : Inport  Port=67
  Data_b05 : Inport  Port=68
  Data_b04 : Inport  Port=69
  Data_b03 : Inport  Port=70
  Data_b02 : Inport  Port=71
  Data_b01 : Inport  Port=72
  Data_b00 : Inport  Port=73
  Write(1b) : Inport  Port=74
  1024x1B_RAM_Simulated : Memory_Blocks_Lib/1024x1B_RAM_Simulated  SystemSampleTime=-1  VariantActivationTime=update diagram  Latency=0  AutoFrameSizeCalculation=off
      settings: LibrarySourceBlock=Memory_Blocks_Lib/Memory_Blocks_Lib/1024x1B_RAM_Simulated
  Bit to Integer Converter2 : simulink/Logic and Bit Operations/Bit to Integer Converter  nbits=16  bitOrder=MSB first  signedOutputValues=Unsigned  outDtype=uint16  outDtypeSigned=Inherit via internal rule
      settings: LibrarySourceBlock=|
      | commutil2/Bit to Integer
      | Converter
  Constant : Constant  Value=0  OutDataTypeStr=boolean
  Data(2B) : Terminator
  Demux2 : Demux  Outputs=8
  Enc_1 : Encoders_Lib/Enc_32  SystemSampleTime=-1  VariantActivationTime=update diagram  Latency=0  AutoFrameSizeCalculation=off
  Enc_32 : Encoders_Lib/Enc_32  SystemSampleTime=-1  VariantActivationTime=update diagram  Latency=0  AutoFrameSizeCalculation=off
  Integer to Bit Converter2 : simulink/Logic and Bit Operations/Integer to Bit Converter  nbits=16  signedInputValues=Unsigned  bitOrder=MSB first  outDtype=boolean
      settings: LibrarySourceBlock=|
      | commutil2/Integer to Bit
      | Converter
  Mux1 : Mux  Inputs=16
  Mux2 : Mux  Inputs=8
  To Workspace2 : ToWorkspace  VariableName=data_bus_vram  SampleTime=-1
      settings: MaxDataPoints=1  Save2DSignal=2-D array (concatenate along first dimension)
  uint_to_bus(byte) : Miscellaneous/uint_to_bus(byte)  SystemSampleTime=-1  VariantActivationTime=update diagram  Latency=0  AutoFrameSizeCalculation=off
  uint_to_bus1 : Miscellaneous/uint_to_bus(word)
      settings: LibrarySourceBlock=Miscellaneous/uint_to_bus
  Video(1000B) : Outport
  b07 : Outport  Port=2
  b06 : Outport  Port=3
  b05 : Outport  Port=4
  b04 : Outport  Port=5
  b03 : Outport  Port=6
  b02 : Outport  Port=7
  b01 : Outport  Port=8
  b00 : Outport  Port=9
  wires:
  1024x1B_RAM_Simulated/1 -> Video(1000B)/1, To Workspace2/1
  X31/1 -> Enc_1/1
  Y28/1 -> Enc_32/4
  X05/1 -> Enc_1/27
  X00/1 -> Enc_1/32
  X01/1 -> Enc_1/31
  Y14/1 -> Enc_32/18
  X17/1 -> Enc_1/15
  CLK/1 -> 1024x1B_RAM_Simulated/4
  Write(1b)/1 -> 1024x1B_RAM_Simulated/2
  Y10/1 -> Enc_32/22
  uint_to_bus1/1 -> 1024x1B_RAM_Simulated/1
  Y12/1 -> Enc_32/20
  Y24/1 -> Enc_32/8
  Y08/1 -> Enc_32/24
  Y30/1 -> Enc_32/2
  Y01/1 -> Enc_32/31
  Y05/1 -> Enc_32/27
  Y11/1 -> Enc_32/21
  Y00/1 -> Enc_32/32
  Y15/1 -> Enc_32/17
  Y04/1 -> Enc_32/28
  Y02/1 -> Enc_32/30
  X28/1 -> Enc_1/4
  X02/1 -> Enc_1/30
  Y27/1 -> Enc_32/5
  X09/1 -> Enc_1/23
  Y17/1 -> Enc_32/15
  X04/1 -> Enc_1/28
  Y16/1 -> Enc_32/16
  Y22/1 -> Enc_32/10
  X06/1 -> Enc_1/26
  Y19/1 -> Enc_32/13
  X12/1 -> Enc_1/20
  X20/1 -> Enc_1/12
  X07/1 -> Enc_1/25
  Y03/1 -> Enc_32/29
  X11/1 -> Enc_1/21
  Y20/1 -> Enc_32/12
  X22/1 -> Enc_1/10
  X13/1 -> Enc_1/19
  X03/1 -> Enc_1/29
  X08/1 -> Enc_1/24
  Y25/1 -> Enc_32/7
  Mux1/1 -> Bit to Integer Converter2/1
  Y31/1 -> Enc_32/1
  Y13/1 -> Enc_32/19
  X10/1 -> Enc_1/22
  X26/1 -> Enc_1/6
  X14/1 -> Enc_1/18
  X27/1 -> Enc_1/5
  X24/1 -> Enc_1/8
  X16/1 -> Enc_1/16
  X15/1 -> Enc_1/17
  X23/1 -> Enc_1/9
  Y23/1 -> Enc_32/9
  X21/1 -> Enc_1/11
  Y18/1 -> Enc_32/14
  X25/1 -> Enc_1/7
  X30/1 -> Enc_1/2
  Constant/1 -> Mux1/1, Mux1/2, Mux1/3, Mux1/4, Mux1/5, Mux1/6
  Y07/1 -> Enc_32/25
  Y09/1 -> Enc_32/23
  Y26/1 -> Enc_32/6
  X29/1 -> Enc_1/3
  Bit to Integer Converter2/1 -> uint_to_bus1/1
  Y21/1 -> Enc_32/11
  Y29/1 -> Enc_32/3
  Y06/1 -> Enc_32/26
  X19/1 -> Enc_1/13
  X18/1 -> Enc_1/14
  Enc_32/5 -> Mux1/16
  Enc_32/4 -> Mux1/15
  Enc_32/3 -> Mux1/14
  Enc_32/2 -> Mux1/13
  Enc_32/1 -> Mux1/12
  Enc_1/5 -> Mux1/11
  Enc_1/4 -> Mux1/10
  Enc_1/3 -> Mux1/9
  Enc_1/2 -> Mux1/8
  Enc_1/1 -> Mux1/7
  Demux2/3 -> b05/1  "b05"
  Demux2/5 -> b03/1  "b03"
  Demux2/6 -> b02/1  "b02"
  Demux2/8 -> b00/1  "b00"
  Integer to Bit Converter2/1 -> Demux2/1
  Demux2/7 -> b01/1  "b01"
  Demux2/4 -> b04/1  "b04"
  Demux2/2 -> b06/1  "b06"
  Demux2/1 -> b07/1  "b07"
  1024x1B_RAM_Simulated/2 -> Data(2B)/1, Integer to Bit Converter2/1
  Data_b02/1 -> Mux2/6
  Data_b01/1 -> Mux2/7
  Data_b00/1 -> Mux2/8
  Data_b03/1 -> Mux2/5
  Data_b04/1 -> Mux2/4
  Data_b07/1 -> Mux2/1
  Data_b05/1 -> Mux2/3
  Data_b06/1 -> Mux2/2
  Mux2/1 -> uint_to_bus(byte)/1
  uint_to_bus(byte)/1 -> 1024x1B_RAM_Simulated/3

== system Computer/Word_Enable27 ==
  note: Word_Enable
  Sel(1b) : Inport
  b07 : Inport  Port=2
  b06 : Inport  Port=3
  b05 : Inport  Port=4
  b04 : Inport  Port=5
  b03 : Inport  Port=6
  b02 : Inport  Port=7
  b01 : Inport  Port=8
  b00 : Inport  Port=9
  Logical Operator{1..8} (8 alike) : Logic  IconShape=distinctive  AllPortsSameDT=off  OutDataTypeStr=boolean
  "b07 " : Outport
  "b06 " : Outport  Port=2
  "b05 " : Outport  Port=3
  "b04 " : Outport  Port=4
  "b03 " : Outport  Port=5
  "b02 " : Outport  Port=6
  "b01 " : Outport  Port=7
  "b00 " : Outport  Port=8
  wires:
  Logical Operator8/1 -> "b07 "/1  "b07"
  Logical Operator3/1 -> "b02 "/1  "b02"
  Logical Operator5/1 -> "b04 "/1  "b04"
  Logical Operator1/1 -> "b01 "/1  "b01"
  Logical Operator6/1 -> "b05 "/1  "b05"
  Logical Operator2/1 -> "b00 "/1  "b00"
  Logical Operator7/1 -> "b06 "/1  "b06"
  Logical Operator4/1 -> "b03 "/1  "b03"
  b00/1 -> Logical Operator2/2
  b01/1 -> Logical Operator1/2
  b02/1 -> Logical Operator3/2
  b03/1 -> Logical Operator4/2
  b04/1 -> Logical Operator5/2
  b05/1 -> Logical Operator6/2
  b06/1 -> Logical Operator7/2
  b07/1 -> Logical Operator8/2
  Sel(1b)/1 -> Logical Operator8/1, Logical Operator7/1, Logical Operator6/1, Logical Operator5/1, Logical Operator4/1, Logical Operator3/1, Logical Operator1/1, Logical Operator2/1

== system Computer/Word_Enable28 ==
  note: Word_Enable
  Sel(1b) : Inport
  b07 : Inport  Port=2
  b06 : Inport  Port=3
  b05 : Inport  Port=4
  b04 : Inport  Port=5
  b03 : Inport  Port=6
  b02 : Inport  Port=7
  b01 : Inport  Port=8
  b00 : Inport  Port=9
  Logical Operator{1..8} (8 alike) : Logic  IconShape=distinctive  AllPortsSameDT=off  OutDataTypeStr=boolean
  "b07 " : Outport
  "b06 " : Outport  Port=2
  "b05 " : Outport  Port=3
  "b04 " : Outport  Port=4
  "b03 " : Outport  Port=5
  "b02 " : Outport  Port=6
  "b01 " : Outport  Port=7
  "b00 " : Outport  Port=8
  wires:
  Logical Operator8/1 -> "b07 "/1  "b07"
  Logical Operator3/1 -> "b02 "/1  "b02"
  Logical Operator5/1 -> "b04 "/1  "b04"
  Logical Operator1/1 -> "b01 "/1  "b01"
  Logical Operator6/1 -> "b05 "/1  "b05"
  Logical Operator2/1 -> "b00 "/1  "b00"
  Logical Operator7/1 -> "b06 "/1  "b06"
  Logical Operator4/1 -> "b03 "/1  "b03"
  b00/1 -> Logical Operator2/2
  b01/1 -> Logical Operator1/2
  b02/1 -> Logical Operator3/2
  b03/1 -> Logical Operator4/2
  b04/1 -> Logical Operator5/2
  b05/1 -> Logical Operator6/2
  b06/1 -> Logical Operator7/2
  b07/1 -> Logical Operator8/2
  Sel(1b)/1 -> Logical Operator8/1, Logical Operator7/1, Logical Operator6/1, Logical Operator5/1, Logical Operator4/1, Logical Operator3/1, Logical Operator1/1, Logical Operator2/1

== system Computer/Word_Enable29 ==
  note: Word_Enable
  Sel(1b) : Inport
  b07 : Inport  Port=2
  b06 : Inport  Port=3
  b05 : Inport  Port=4
  b04 : Inport  Port=5
  b03 : Inport  Port=6
  b02 : Inport  Port=7
  b01 : Inport  Port=8
  b00 : Inport  Port=9
  Logical Operator{1..8} (8 alike) : Logic  IconShape=distinctive  AllPortsSameDT=off  OutDataTypeStr=boolean
  "b07 " : Outport
  "b06 " : Outport  Port=2
  "b05 " : Outport  Port=3
  "b04 " : Outport  Port=4
  "b03 " : Outport  Port=5
  "b02 " : Outport  Port=6
  "b01 " : Outport  Port=7
  "b00 " : Outport  Port=8
  wires:
  Logical Operator8/1 -> "b07 "/1  "b07"
  Logical Operator3/1 -> "b02 "/1  "b02"
  Logical Operator5/1 -> "b04 "/1  "b04"
  Logical Operator1/1 -> "b01 "/1  "b01"
  Logical Operator6/1 -> "b05 "/1  "b05"
  Logical Operator2/1 -> "b00 "/1  "b00"
  Logical Operator7/1 -> "b06 "/1  "b06"
  Logical Operator4/1 -> "b03 "/1  "b03"
  b00/1 -> Logical Operator2/2
  b01/1 -> Logical Operator1/2
  b02/1 -> Logical Operator3/2
  b03/1 -> Logical Operator4/2
  b04/1 -> Logical Operator5/2
  b05/1 -> Logical Operator6/2
  b06/1 -> Logical Operator7/2
  b07/1 -> Logical Operator8/2
  Sel(1b)/1 -> Logical Operator8/1, Logical Operator7/1, Logical Operator6/1, Logical Operator5/1, Logical Operator4/1, Logical Operator3/1, Logical Operator1/1, Logical Operator2/1
